simulink model "testrig_Linkage_Shock"  (R2025a)
settings: Solver=ode23t  StartTime=0.0  StopTime=16  RelTol=1e-3  AbsTol=1e-3  EnableMultiTasking=on
undefined symbols (not defined in the file): VDatabase, X, Y, Z
libraries: sm_lib x5, nesl_utility x3, Damper_Linear x2, fl_lib x2, simulink x2, Linkage_Shock x2, Spring_Linear x2
Description:
  | Copyright 2025 The MathWorks, Inc.
settings Model: Creator=smiller  LastModifiedBy=smiller
settings SolverCC: AutoScaleAbsTol=off  AlgebraicLoopSolver=TrustRegion  MaxZcPerStep=1.0
settings DataIOCC: LimitDataPoints=on  MaxDataPoints=10000
settings OptimizationCC: LifeSpan=inf
settings DebuggingCC: UnconnectedInputMsg=warning  UnconnectedOutputMsg=warning  UnconnectedLineMsg=warning  AllowSymbolicDim=off  SFUnexpectedBacktrackingDiag=warning  SFNoUnconditionalDefaultTransitionDiag=warning  SFExecutionAtInitializationDiag=none  ArithmeticOperatorsInVariantConditions=warning
settings ModelReferenceCC: EnableRefExpFcnMdlSchedulingChecks=on
settings SFSimCC: SimUseLocalCustomCode=off  CustomCodeUndefinedFunction=UseInterfaceOnly
settings RTWCC: RTWUseLocalCustomCode=off  GPUComputeCapability=3.5  DLArmComputeVersion=19.05
settings CodeAppCC: StateflowObjectComments=on
settings GRTTargetCC: TargetLangStandard=C89/C90 (ANSI)
settings ConfigComp: CovMetricSettings=dw  CovSaveCumulativeToWorkspaceVar=on  CovSaveSingleToWorkspaceVar=on  CovExternalEMLEnable=off  CovSFcnEnable=off
settings SimscapeCC: SimscapeLogType=all  SimscapeLogSimulationStatistics=on  SimscapeLogDataHistory=10000.0
settings DiagnosticsConfigSet: SimMechanicsJointTargetOverSpecification=warning
settings ExplorerConfigSet: InternalSimMechanicsExplorerSettings="<ExplorerConfiguration><canonicalview>default</canonicalview><AnimationSetting><BasePlaybackSpeed>1.0</BasePlaybackSpeed><PlaybackSpeedFactor>1.0</PlaybackSpeedFactor></AnimationSetting><TilePanel><TileInfo><Tiles Columns=\"1\" Count=\"1\" Rows=\"1\"><Column Weight=\"1\"/><Row Weight=\"1\"/><Tile Height=\"1\" Width=\"1\" X=\"0\" Y=\"0\"/></Tiles></TileInfo><SceneInfo><SceneViewer><BGColor><R>1</R><G>1</G><B>1</B></BGColor><Camera><DoPerspective>off</DoPerspective><Position><X>0.149999996270014591</X><Y>-0.999999999792783312</Y><Z>0.271043833746434037</Z></Position><Center><X>0.149999996270014591</X><Y>2.07216632741591411e-10</Y><Z>0.271043833746434037</Z></Center><Up><X>0</X><Y>-0</Y><Z>1</Z></Up><ViewLimDist>1</ViewLimDist><YLim>0.304925158321857459</YLim><XLim>0.420940454249028817</XLim></Camera></SceneViewer></SceneInfo></TilePanel><MechEditorPanel><Cameras/><GfxPanelCameraMap/><VideoCreator><PlaybackSpeedRatio>1.0</PlaybackSpeedRatio><FrameRate>30</FrameRate><VideoFormat>Motion JPEG AVI</VideoFormat><FrameSize>auto</FrameSize></VideoCreator></MechEditorPanel></ExplorerConfiguration>"

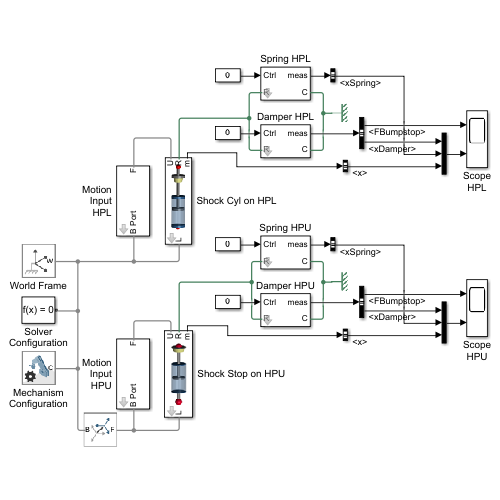
[thumbnail: Simulink's stored preview of the top-level diagram]
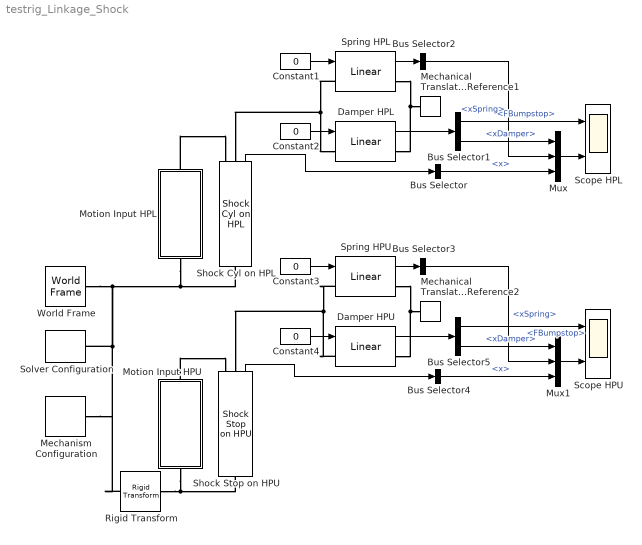
== system testrig_Linkage_Shock ==
  Bus Selector : BusSelector  OutputSignals=x
  Bus Selector1 : BusSelector  OutputSignals=FBumpstop,xDamper
  Bus Selector2 : BusSelector  OutputSignals=xSpring
  Bus Selector3 : BusSelector  OutputSignals=xSpring
  Bus Selector4 : BusSelector  OutputSignals=x
  Bus Selector5 : BusSelector  OutputSignals=FBumpstop,xDamper
  Constant{1..4} (4 alike) : Constant  Value=0
  Damper HPL : Damper_Linear/Linear  VariantControl=Linear  dam_b=VDatabase.Damper.Sedan_Hamba_Linear_A1.Damping.d.Value  hp_dpr_top=VDatabase.Damper.Sedan_Hamba_Linear_A1.Damping.sTop.Value  hp_dpr_bot=VDatabase.Damper.Sedan_Hamba_Linear_A1.Damping.sBottom.Value  bs_lim_upper=VDatabase.Damper.Sedan_Hamba_Linear_A1.Endstop.xMax.Value  bs_lim_lower=VDatabase.Damper.Sedan_Hamba_Linear_A1.Endstop.xMin.Value  bs_k_upper=VDatabase.Damper.Sedan_Hamba_Linear_A1.Endstop.KxMax.Value  bs_k_lower=VDatabase.Damper.Sedan_Hamba_Linear_A1.Endstop.KxMin.Value  bs_b_upper=VDatabase.Damper.Sedan_Hamba_Linear_A1.Endstop.dxMax.Value  bs_b_lower=VDatabase.Damper.Sedan_Hamba_Linear_A1.Endstop.dxMin.Value  bs_region=VDatabase.Damper.Sedan_Hamba_Linear_A1.Endstop.xTransition.Value
  Damper HPU : Damper_Linear/Linear  VariantControl=Linear  dam_b=VDatabase.Damper.Sedan_Hamba_Linear_A1.Damping.d.Value  hp_dpr_top=VDatabase.Damper.Sedan_Hamba_Linear_A1.Damping.sTop.Value  hp_dpr_bot=VDatabase.Damper.Sedan_Hamba_Linear_A1.Damping.sBottom.Value  bs_lim_upper=VDatabase.Damper.Sedan_Hamba_Linear_A1.Endstop.xMax.Value  bs_lim_lower=VDatabase.Damper.Sedan_Hamba_Linear_A1.Endstop.xMin.Value  bs_k_upper=VDatabase.Damper.Sedan_Hamba_Linear_A1.Endstop.KxMax.Value  bs_k_lower=VDatabase.Damper.Sedan_Hamba_Linear_A1.Endstop.KxMin.Value  bs_b_upper=VDatabase.Damper.Sedan_Hamba_Linear_A1.Endstop.dxMax.Value  bs_b_lower=VDatabase.Damper.Sedan_Hamba_Linear_A1.Endstop.dxMin.Value  bs_region=VDatabase.Damper.Sedan_Hamba_Linear_A1.Endstop.xTransition.Value
  Mechanical Translational Reference1 : fl_lib/Mechanical/Translational Elements/Mechanical Translational Reference
  Mechanical Translational Reference2 : fl_lib/Mechanical/Translational Elements/Mechanical Translational Reference
  Mechanism Configuration : sm_lib/Utilities/Mechanism Configuration  UniformGravity=Constant  GravityVector=[0 0 -9.80665]  GravityVectorUnits=m/s^2  LinearizationDelta=0.001  JointModeTransitionNonlinearIterations=2
  Motion Input HPL : Subsystem  mask{hp_top=VDatabase.Linkage.DoubleWishbone_Sedan_Hamba_f.Shock.sTop.Value, hp_bot=VDatabase.Linkage.DoubleWishbone_Sedan_Hamba_f.Shock.sBottom.Value, xMax=VDatabase.Linkage.DoubleWishbone_Sedan_Hamba_f.Endstop.xMax.Value, xMin=VDatabase.Linkage.DoubleWishbone_Sedan_Hamba_f.Endstop.xMin.Value, xPen=5e-3}
      mask prompts: hp_top "HP Top"; hp_bot "HP Bottom"; xMax "Upper Lim"; xMin "Lower Lim"; xPen "Penetration"
      mask init:
      | xStart = sqrt(sum((hp_top-hp_bot).^2));
  Motion Input HPU : Subsystem  mask{hp_top=VDatabase.Linkage.DoubleWishbone_Sedan_Hamba_f.Shock.sTop.Value, hp_bot=VDatabase.Linkage.DoubleWishbone_Sedan_Hamba_f.Shock.sBottom.Value, xMax=VDatabase.Linkage.DoubleWishbone_Sedan_Hamba_f.Endstop.xMax.Value, xMin=VDatabase.Linkage.DoubleWishbone_Sedan_Hamba_f.Endstop.xMin.Value, xPen=5e-3}
      mask prompts: hp_top "HP Top"; hp_bot "HP Bottom"; xMax "Upper Lim"; xMin "Lower Lim"; xPen "Penetration"
      mask init:
      | xStart = sqrt(sum((hp_top-hp_bot).^2));
  Mux : Mux  Inputs=3
  Mux1 : Mux  Inputs=3
  Rigid Transform : sm_lib/Frames and Transforms/Rigid Transform  RotationMethod=None  FollAlignAxisA=+X  BaseAlignAxisA=+Y  FollAlignAxisB=+Y  BaseAlignAxisB=+Z  RotationStandardAxis=+Z  RotationAngle=0  RotationAngleUnits=deg  RotationArbitraryAxis=[0 0 1]  RotationSequenceAxes=FollowerAxes  RotationSequence=XYX  RotationSequenceAngles=[0 0 0]  RotationSequenceAnglesUnits=deg  RotationMatrix=[1 0 0;0 1 0;0 0 1]  Quaternion=[1 0 0 0]  TranslationMethod=StandardAxis  TranslationCartesianOffset=[0 0 0]  TranslationCartesianOffsetUnits=m  TranslationStandardAxis=+X  TranslationStandardOffset=0.3  TranslationStandardOffsetUnits=m  TranslationROffset=0  TranslationROffsetUnits=m  TranslationThetaOffset=0  TranslationThetaOffsetUnits=deg  TranslationZOffset=0  TranslationZOffsetUnits=m
  Scope HPL : Scope  NumInputPorts=2
      settings: ActiveDisplayYMinimum=-5691.75402  ActiveDisplayYMaximum=5689.27715
  Scope HPU : Scope  NumInputPorts=2
      settings: ActiveDisplayYMinimum=-5691.75402  ActiveDisplayYMaximum=5689.27715
  Shock Cyl on HPL : Linkage_Shock/Shock Cyl on HPL  shock_pist_mass=VDatabase.Linkage.DoubleWishbone_Sedan_Hamba_f.Shock.mPiston.Value  shock_cyl_mass=VDatabase.Linkage.DoubleWishbone_Sedan_Hamba_f.Shock.mCylinder.Value  hp_spr_top=VDatabase.Linkage.DoubleWishbone_Sedan_Hamba_f.Shock.sTop.Value  hp_spr_bot=VDatabase.Linkage.DoubleWishbone_Sedan_Hamba_f.Shock.sBottom.Value  up_lim_bumpstop=VDatabase.Linkage.DoubleWishbone_Sedan_Hamba_f.Endstop.xMax.Value  low_lim_bumpstop=VDatabase.Linkage.DoubleWishbone_Sedan_Hamba_f.Endstop.xMin.Value  clr_conn_shock=Visual.hp.clr  opc_conn_shock=Visual.hp.opc  size_conn_shock=Visual.hp.rad  clr_shock_cyl=Visual.clr.blue  opc_shock_cyl=Visual.part.opc  radius_shock_cyl=0.05  clr_shock_piston=Visual.clr.gray  opc_shock_piston=Visual.part.opc  clr_shock_bumpstop=Visual.clr.yellowpale  opc_shock_bumpstop=Visual.part.opc  deadvol_len_shock_cyl=Visual.Shock.dead_length  piston_len_shock=Visual.Shock.piston.len  cyl_cap_len_shock=Visual.Shock.cap.len  bumpstop_len_shock=Visual.Shock.bumpstop.len
  Shock Stop on HPU : Linkage_Shock/Shock Stop on HPU  shock_pist_mass=VDatabase.Linkage.DoubleWishbone_Sedan_Hamba_f.Shock.mPiston.Value  shock_cyl_mass=VDatabase.Linkage.DoubleWishbone_Sedan_Hamba_f.Shock.mCylinder.Value  hp_spr_top=VDatabase.Linkage.DoubleWishbone_Sedan_Hamba_f.Shock.sTop.Value  hp_spr_bot=VDatabase.Linkage.DoubleWishbone_Sedan_Hamba_f.Shock.sBottom.Value  up_lim_bumpstop=VDatabase.Linkage.DoubleWishbone_Sedan_Hamba_f.Endstop.xMax.Value  low_lim_bumpstop=VDatabase.Linkage.DoubleWishbone_Sedan_Hamba_f.Endstop.xMin.Value  clr_conn_shock=Visual.hp.clr  opc_conn_shock=Visual.hp.opc  size_conn_shock=Visual.hp.rad  clr_shock_cyl=Visual.clr.blue  opc_shock_cyl=Visual.part.opc  radius_shock_cyl=0.05  clr_shock_piston=Visual.clr.gray  opc_shock_piston=Visual.part.opc  clr_shock_bumpstop=Visual.clr.yellowpale  opc_shock_bumpstop=Visual.part.opc  deadvol_len_shock_cyl=Visual.Shock.dead_length  piston_len_shock=Visual.Shock.piston.len  cyl_cap_len_shock=Visual.Shock.cap.len  bumpstop_len_shock=Visual.Shock.bumpstop.len
  Solver Configuration : nesl_utility/Solver Configuration  PhysicalDomain=network_engine_domain  SubClassName=solver  LeftPortType=input  RightPortType=generic  Tones=[]  Harmonics=[]  SimulateNoise=off  Profile=off  UseLocalSampling=off  EnableSwitchedLinearOptims=on  FrequencyDomain=off  UseCCode=off  RelTol=0.001  AbsTol=1e-06  MinStep=1e-09  ToWorkspace=off  RevertToSquareIcSolve=off  NumHomotopyIterations=100  PhasorMode=off  PhasorModeNumHarmonics=1  ConsistencySolver=NEWTON_XTOL_AFTER_FTOL  IndexReductionMethod=DerivativeReplacement  DoDC=off  ResidualTolerance=1e-09  ConsistencyTolSource=GLOBAL  ConsistencyAbsTol=0.001  ConsistencyRelTol=0.001  ConsistencyTolFactor=0.001  UseLocalSolver=off  LocalSolverChoice=NE_BACKWARD_EULER_ADVANCER  ResolveIndetEquations=on  FunctionEvalNumThread=1  LocalSolverSampleTime=0.001  DoFixedCost=off  MaxNonlinIter=3  MaxModeIter=2  ComputeImpulses=off  ImpulseIterations=2  LinearAlgebra=Sparse  LinearAlgebraNumThread=0  EquationFormulation=NE_TIME_EF  DelaysMemoryBudget=1024  AutomaticFiltering=on  FilteringTimeConstant=0.001  PartitionStorageMethod=AS_NEEDED  PartitionMemoryBudget=1024  PartitionMethod=FAST  MultibodyUseLocalSolver=off  MultibodyLocalSolverChoice=ODE1  MultibodyLocalSolverSampleTime=0.001
  Spring HPL : Spring_Linear/Linear  VariantControl=Linear  spr_def0=VDatabase.Spring.Sedan_Hamba_Linear_A1.xPreload.Value  spr_frc0=VDatabase.Spring.Sedan_Hamba_Linear_A1.fPreload.Value  spr_k=VDatabase.Spring.Sedan_Hamba_Linear_A1.K.Value  spr_hp_top=VDatabase.Spring.Sedan_Hamba_Linear_A1.sTop.Value  spr_hp_bot=VDatabase.Spring.Sedan_Hamba_Linear_A1.sBottom.Value
  Spring HPU : Spring_Linear/Linear  VariantControl=Linear  spr_def0=VDatabase.Spring.Sedan_Hamba_Linear_A1.xPreload.Value  spr_frc0=VDatabase.Spring.Sedan_Hamba_Linear_A1.fPreload.Value  spr_k=VDatabase.Spring.Sedan_Hamba_Linear_A1.K.Value  spr_hp_top=VDatabase.Spring.Sedan_Hamba_Linear_A1.sTop.Value  spr_hp_bot=VDatabase.Spring.Sedan_Hamba_Linear_A1.sBottom.Value
  World Frame : sm_lib/Frames and Transforms/World Frame
  wires:
  Spring HPL/1 -> Bus Selector2/1
  Constant1/1 -> Spring HPL/1
  Shock Cyl on HPL/1 -> Bus Selector/1
  Constant2/1 -> Damper HPL/1
  Damper HPL/1 -> Bus Selector1/1
  Bus Selector1/1 -> Scope HPL/1  "<FBumpstop>"
  Bus Selector/1 -> Mux/3  "<x>"
  Bus Selector1/2 -> Mux/1  "<xDamper>"
  Mux/1 -> Scope HPL/2
  Bus Selector2/1 -> Mux/2  "<xSpring>"
  Damper HPU/1 -> Bus Selector5/1
  Constant4/1 -> Damper HPU/1
  Constant3/1 -> Spring HPU/1
  Spring HPU/1 -> Bus Selector3/1
  Bus Selector3/1 -> Mux1/2  "<xSpring>"
  Mux1/1 -> Scope HPU/2
  Bus Selector5/2 -> Mux1/1  "<xDamper>"
  Bus Selector4/1 -> Mux1/3  "<x>"
  Bus Selector5/1 -> Scope HPU/1  "<FBumpstop>"
  Shock Stop on HPU/1 -> Bus Selector4/1
  connections:
  Motion Input HPL/LConn1 -- Mechanism Configuration/RConn1 -- Rigid Transform/LConn1 -- Solver Configuration/RConn1 -- World Frame/RConn1 -- Shock Cyl on HPL/LConn1
  Motion Input HPL/RConn1 -- Shock Cyl on HPL/RConn2
  Spring HPL/LConn1 -- Shock Cyl on HPL/RConn1 -- Damper HPL/LConn1
  Spring HPL/RConn1 -- Damper HPL/RConn1 -- Mechanical Translational Reference1/LConn1
  Rigid Transform/RConn1 -- Shock Stop on HPU/LConn1 -- Motion Input HPU/LConn1
  Motion Input HPU/RConn1 -- Shock Stop on HPU/RConn2
  Damper HPU/LConn1 -- Spring HPU/LConn1 -- Shock Stop on HPU/RConn1
  Spring HPU/RConn1 -- Damper HPU/RConn1 -- Mechanical Translational Reference2/LConn1

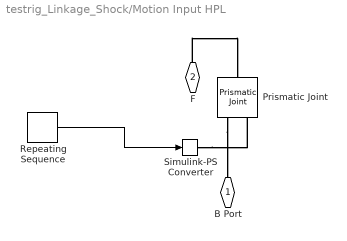
== system testrig_Linkage_Shock/Motion Input HPL ==
  Prismatic Joint : sm_lib/Joints/Prismatic Joint  JointMode=Normal  CompositeWrenchDir=FollowerOnBase  CompositeWrenchFrame=BaseFrame  SenseConstraintForce=off  SenseConstraintTorque=off  SenseTotalForce=off  SenseTotalTorque=off  PositionTargetSpecify=on  PositionTargetPriority=High  PositionTargetValue=xStart  PositionTargetValueUnits=m  VelocityTargetSpecify=off  VelocityTargetPriority=High  VelocityTargetValue=0  VelocityTargetValueUnits=m/s  EquilibriumPosition=0  EquilibriumPositionUnits=m  SpringStiffness=0  SpringStiffnessUnits=N/m  DampingCoefficient=0  DampingCoefficientUnits=N/(m/s)  LowerLimitSpecify=off  LowerLimitBound=-1  LowerLimitBoundUnits=m  LowerLimitStiffness=1e6  LowerLimitStiffnessUnits=N/m  LowerLimitDamping=1e3  LowerLimitDampingUnits=N/(m/s)  LowerLimitTransitionRegionWidth=1e-4  LowerLimitTransitionRegionWidthUnits=m  UpperLimitSpecify=off  UpperLimitBound=1  UpperLimitBoundUnits=m  UpperLimitStiffness=1e6  UpperLimitStiffnessUnits=N/m  UpperLimitDamping=1e3  UpperLimitDampingUnits=N/(m/s)  UpperLimitTransitionRegionWidth=1e-4  UpperLimitTransitionRegionWidthUnits=m  TorqueActuationMode=ComputedTorque  MotionActuationMode=InputMotion  SensePosition=off  SenseVelocity=off  SenseAcceleration=off  SenseTorqueForce=off  SenseLowerLimitTorqueForce=off  SenseUpperLimitTorqueForce=off
  Repeating Sequence : simulink/Sources/Repeating Sequence  rep_seq_t=[0 2 4 6 8 10 12 14 16]  rep_seq_y=[0 0 xMax xMax+xPen 0 xMin xMin-xPen 0 0]+xStart
  Simulink-PS Converter : nesl_utility/Simulink-PS Converter  PhysicalDomain=network_engine_domain  SubClassName=ps_input  LeftPortType=input  RightPortType=output  PseudoPeriodic=off  Frequencies=[]  NoiseDistribution=none  NoiseParameters=[]  Unit=m  AffineConversion=off  FilteringAndDerivatives=filter  SimscapeFilterOrder=2  InputFilterTimeConstant=0.1  UdotUserProvided=0
  B Port : PMIOPort  Side=Left
  F : PMIOPort  Port=2  Side=Right
  wires:
  Repeating Sequence/1 -> Simulink-PS Converter/1
  connections:
  Simulink-PS Converter/RConn1 -- Prismatic Joint/LConn2
  Prismatic Joint/LConn1 -- B Port/RConn1
  F/RConn1 -- Prismatic Joint/RConn1

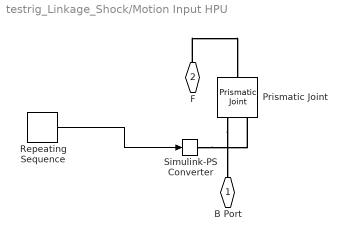
== system testrig_Linkage_Shock/Motion Input HPU ==
  Prismatic Joint : sm_lib/Joints/Prismatic Joint  JointMode=Normal  CompositeWrenchDir=FollowerOnBase  CompositeWrenchFrame=BaseFrame  SenseConstraintForce=off  SenseConstraintTorque=off  SenseTotalForce=off  SenseTotalTorque=off  PositionTargetSpecify=on  PositionTargetPriority=High  PositionTargetValue=xStart  PositionTargetValueUnits=m  VelocityTargetSpecify=off  VelocityTargetPriority=High  VelocityTargetValue=0  VelocityTargetValueUnits=m/s  EquilibriumPosition=0  EquilibriumPositionUnits=m  SpringStiffness=0  SpringStiffnessUnits=N/m  DampingCoefficient=0  DampingCoefficientUnits=N/(m/s)  LowerLimitSpecify=off  LowerLimitBound=-1  LowerLimitBoundUnits=m  LowerLimitStiffness=1e6  LowerLimitStiffnessUnits=N/m  LowerLimitDamping=1e3  LowerLimitDampingUnits=N/(m/s)  LowerLimitTransitionRegionWidth=1e-4  LowerLimitTransitionRegionWidthUnits=m  UpperLimitSpecify=off  UpperLimitBound=1  UpperLimitBoundUnits=m  UpperLimitStiffness=1e6  UpperLimitStiffnessUnits=N/m  UpperLimitDamping=1e3  UpperLimitDampingUnits=N/(m/s)  UpperLimitTransitionRegionWidth=1e-4  UpperLimitTransitionRegionWidthUnits=m  TorqueActuationMode=ComputedTorque  MotionActuationMode=InputMotion  SensePosition=off  SenseVelocity=off  SenseAcceleration=off  SenseTorqueForce=off  SenseLowerLimitTorqueForce=off  SenseUpperLimitTorqueForce=off
  Repeating Sequence : simulink/Sources/Repeating Sequence  rep_seq_t=[0 2 4 6 8 10 12 14 16]  rep_seq_y=[0 0 xMax xMax+xPen 0 xMin xMin-xPen 0 0]+xStart
  Simulink-PS Converter : nesl_utility/Simulink-PS Converter  PhysicalDomain=network_engine_domain  SubClassName=ps_input  LeftPortType=input  RightPortType=output  PseudoPeriodic=off  Frequencies=[]  NoiseDistribution=none  NoiseParameters=[]  Unit=m  AffineConversion=off  FilteringAndDerivatives=filter  SimscapeFilterOrder=2  InputFilterTimeConstant=0.1  UdotUserProvided=0
  B Port : PMIOPort  Side=Left
  F : PMIOPort  Port=2  Side=Right
  wires:
  Repeating Sequence/1 -> Simulink-PS Converter/1
  connections:
  F/RConn1 -- Prismatic Joint/RConn1
  Prismatic Joint/LConn1 -- B Port/RConn1
  Simulink-PS Converter/RConn1 -- Prismatic Joint/LConn2
